simulink model "control_LQR_subsystem"  (R2023b)
settings: Solver=VariableStepAuto  StartTime=0.0  StopTime=10.0  RelTol=1e-3
settings Model: Creator=tiwan  LastModifiedBy=tiwan

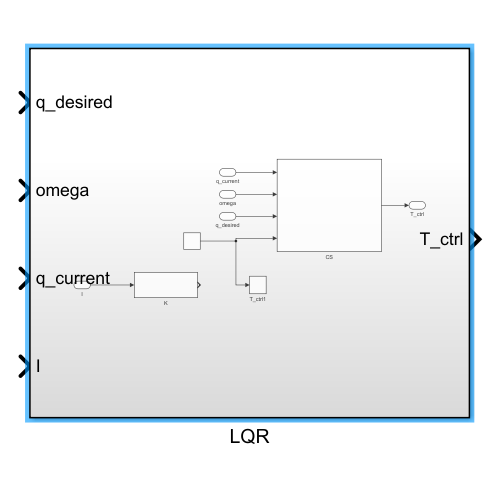
[thumbnail: Simulink's stored preview of the top-level diagram]
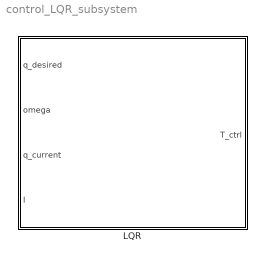
== system control_LQR_subsystem ==
  LQR : Subsystem

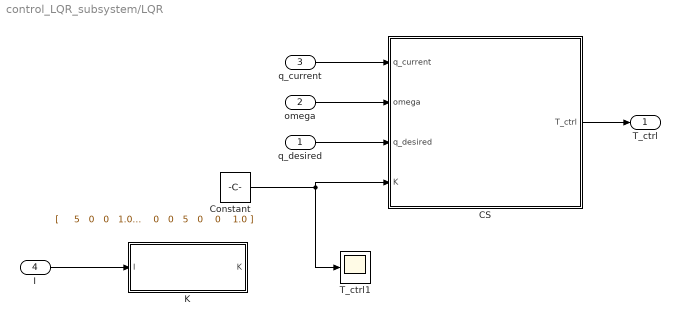
== system control_LQR_subsystem/LQR ==
  q_desired : Inport
  omega : Inport  Port=2
  q_current : Inport  Port=3
  I : Inport  Port=4
  CS : MATLAB Function  TreatAsAtomicUnit=on
  Constant : Constant  Value=|
      | [
      |     5   0   0   1.0  0    0;
      |     0   5   0   0    1.0  0;
      |     0   0   5   0    0    1.0
      | ]
  K : MATLAB Function  TreatAsAtomicUnit=on
  T_ctrl1 : Scope
  T_ctrl : Outport
  wires:
  q_desired/1 -> CS/3(q_desired)
  omega/1 -> CS/2(omega)
  q_current/1 -> CS/1(q_current)
  CS/1(T_ctrl) -> T_ctrl/1
  I/1 -> K/1(I)
  Constant/1 -> CS/4(K), T_ctrl1/1

== matlab function control_LQR_subsystem/LQR/CS ==
  data: q_current input; T_ctrl output; omega input; q_desired input; K input
function T_ctrl = lqr_attitude_control(q_current, omega,q_desired, K)
% Inputs:
%   q_current: [4x1] current quaternion
%   omega:     [3x1] angular velocity
%   q_desired: [4x1] desired quaternion
%   K:         [3x6] LQR gain matrix

% Normalize quaternions (important for numerical stability)
q_current = q_current / norm(q_current);
q_desired = q_desired / norm(q_desired);

% Quaternion error: q_err = q_desired ⊗ q_current⁻¹
q_conj = [q_current(1); -q_current(2:4)];
q_err = quatmultiply(q_desired', q_conj')';  % result is 4x1

% Use only vector part of q_err (proportional part)
delta_q = q_err(2:4);  % 3x1

% LQR control law
x = [delta_q; omega];    % 6x1
T_ctrl = -K * x;         % 3x1 torque output

end

== matlab function control_LQR_subsystem/LQR/K ==
  data: K output; I input
function K = computeK_manual(I)
% Fully Simulink-compatible LQR gain using Riccati iteration, no inv()

% Output definition
K = zeros(3,6);

% Validate input inertia
if any(size(I) ~= [3, 3])
    return;
end

% A, B matrices
A = [zeros(3), 0.5 * eye(3);
     zeros(3), zeros(3)];
B = [zeros(3);
     I \ eye(3)];  % Same as inv(I) * I_identity

% LQR weights
Q = diag([100, 100, 100, 5, 5, 5]);
R = 0.1 * eye(3);

% Riccati gradient descent
S = Q;
alpha = 1e-3;
max_iter = 500;
tol = 1e-4;

for i = 1:max_iter
    BT_S = B' * S;
    E = A' * S + S * A - S * B * (R \ BT_S) + Q;
    
    if norm(E, 'fro') < tol
        break;
    end
    
    S = S - alpha * E;
end

% Final LQR gain
K = R \ (B' * S);
end
